simulink model "AC_L16_sim1"  (R2017b)
settings: Solver=VariableStepAuto  StartTime=0.0  StopTime=t_stop  RelTol=1e-3
values from neighbouring files (symbols this model uses):
  da = 0    [AC_L15_Example1.m]    (also in AC_L15_Example2.m = 1; AC_L16_1.m = 1; AC_L16_2.m)
  dy = 0    [AC_L15_Example1.m]    (also in AC_L15_Example2.m; AC_L16_1.m; AC_L16_2.m)
  rho = 0    [AC_L15_Example2.m]    (also in AC_L16_1.m)
libraries: simulink x1
settings Model: Creator=hantao.li  LastModifiedBy=hantao.li

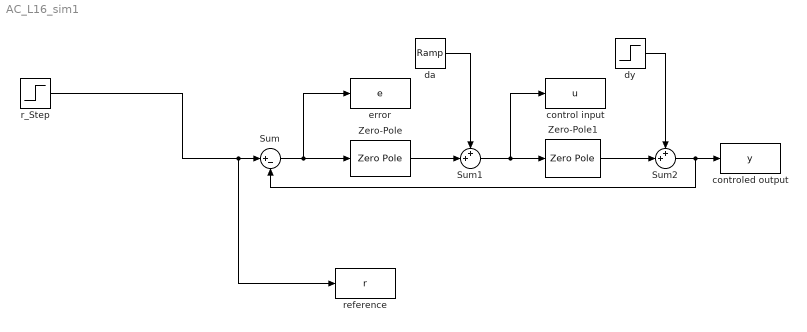
== system AC_L16_sim1 ==
  Sum : Sum  Inputs=|+-
  Sum1 : Sum  Inputs=++|
  Sum2 : Sum  Inputs=++|
  Zero-Pole : ZeroPole  Zeros=[-0.19]  Poles=[0 -0.01967]  Gain=[1.0351]
  Zero-Pole1 : ZeroPole  Zeros=[]  Poles=[-10 -5]  Gain=[100]
  control input : ToWorkspace  VariableName=u  SaveFormat=Timeseries  SampleTime=-1
  controled output : ToWorkspace  VariableName=y  SaveFormat=Timeseries  SampleTime=-1
  da : simulink/Sources/Ramp  slope=da  start=0  X0=0
  dy : Step  Time=0  After=dy  SampleTime=0
  error : ToWorkspace  VariableName=e  SaveFormat=Timeseries  SampleTime=-1
  r_Step : Step  Time=0  After=rho  SampleTime=0
  reference : ToWorkspace  VariableName=r  SaveFormat=Timeseries  SampleTime=-1
  wires:
  r_Step/1 -> reference/1, Sum/1
  Sum/1 -> Zero-Pole/1, error/1
  Zero-Pole/1 -> Sum1/2
  da/1 -> Sum1/1
  Sum1/1 -> Zero-Pole1/1, control input/1
  Zero-Pole1/1 -> Sum2/2
  dy/1 -> Sum2/1
  Sum2/1 -> Sum/2, controled output/1
